simulink model "twa_test"  (R2016a)
settings: Solver=ode8  StartTime=0.0  StopTime=inf  FixedStep=dt  RelTol=1e-3
PreLoadFcn:
  | addpath('d:\Projects\TwistedWireActuator\TWA_parallel_control\init_func')
InitFcn:
  | init_main_twa
  | init_scopes
  | init_twa_homing
  | init_twa_wires
undefined symbols (not defined in the file or in its folder): do_quintic, dt, enc_res_vec, gear_rat_vec, kd_twa, ki_twa, kp_twa, manual_cur, meas_twa_len, N_velocity, pid_mode, pot_volt, q_des, quintic_tf, reset_integ, Signed, vel_filter_coeffs, velmex_pitch, wire_delta, wire_rad
libraries: xpcsensoraylib x4, slrtlib x3, simulink x2, dspswit3 x1
CloseFcn:
  | rtwprivate ssgencode ModelCloseRequest acrochordidae_v1
settings Model: Creator=Roger  LastModifiedBy=ahronoez
settings SolverCC: EnableConcurrentExecution=on
settings DataIOCC: SaveFormat=StructureWithTime  SignalLoggingSaveFormat=ModelDataLogs
settings OptimizationCC: BlockReduction=off  OptimizeBlockIOStorage=off  BufferReuse=off  GlobalBufferReuse=off  ExpressionFolding=off  ExpressionDepthLimit=2147483647  LocalBlockOutputs=off  InitFltsAndDblsToZero=on
settings DebuggingCC: UnderspecifiedInitializationDetection=Classic  MergeDetectMultiDrivingBlocksExec=none  SolverPrmCheckMsg=warning  FcnCallInpInsideContextMsg=UseLocalSettings  StateNameClashWarn=warning
settings HardwareCC: ProdBitPerPointer=32  ProdLargestAtomicFloat=None  ProdWordSize=32  ProdLongLongMode=on  ProdHWDeviceType=Generic->32-bit x86 compatible
settings ModelReferenceCC: PropagateSignalLabelsOutOfModel=off
settings SFSimCC: SimParseCustomCode=off
settings RTWCC: SystemTargetFile=slrt.tlc  TLCOptions=-aSLRTFTZOFF=1  TemplateMakefile=slrt_default_tmf  Description=Simulink Real-Time  GenerateReport=on  RTWCompilerOptimization=Custom  RTWCustomCompilerOptimizations=/arch-IA32
settings SimulinkRealTimeCC: xPCisDownloadable=off
settings ConfigComp: CovModelRefEnable=Off

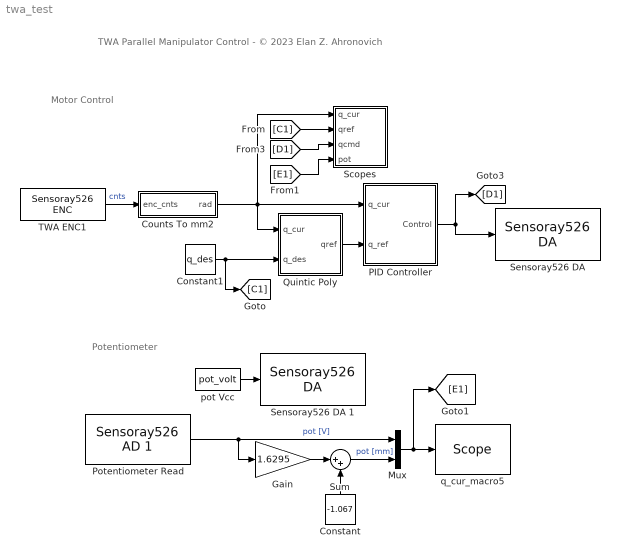
== system twa_test ==
  note: Motor Control
  note: Potentiometer
  note: TWA Parallel Manipulator Control - © 2023 Elan Z. Ahronovich
  Constant : Constant  Value=-1.067
  Constant1 : Constant  Value=q_des
  Counts To mm2 : Subsystem
  Gain : Gain  Gain=1.6295
  Mux : Mux  Inputs=2
  PID Controller : Subsystem
  Potentiometer Read : xpcsensoraylib/A//D/Sensoray526 AD 1  channel=[1]  sampletime=0.001  baseaddress1=0x340  baseaddress2=0
  Quintic Poly : Subsystem
  Scopes : Subsystem
  "Sensoray526 DA " : xpcsensoraylib/D//A/Sensoray526 DA   channel=[4]  reset=[0]  initial=[0]  sampletime=0.001  baseaddress1=0x2c0  baseaddress2=0
  Sensoray526 DA 1 : xpcsensoraylib/D//A/Sensoray526 DA   channel=[2]  reset=[0]  initial=[0]  sampletime=0.001  baseaddress1=0x340  baseaddress2=0
  Sum : Sum  Inputs=|++
  TWA ENC1 : xpcsensoraylib/Encoder/Sensoray526 ENC   channel=4  index=None  resetval=0  initval=0  range=Signed +-2^23  speed=4x  sampletime=dt  baseaddress=0x2c0
  pot Vcc : Constant  Value=pot_volt  SampleTime=-1
  q_cur_macro5 : slrtlib/Displays and Logging/Scope   scopeno=2  scopetype=Target  autostart=on  viewmode=Numerical  formatstr='%0.6f,%0.6f'  grid=on  ylimits=[0,0]  nosamples=125  noprepostsamples=0  interleave=1  triggermode=FreeRun  triggersignal=1  trigsignalfromport=off  triggerlevel=0.0  triggerslope=Either  triggerscope=1  triggersample=0  filename=data.dat  mode=Lazy  writesize=512  autorestart=off  dynamicfilemode=off  maxwritefilesize=512*1024^2
  wires:
  PID Controller/1(Control) -> "Sensoray526 DA "/1, [D1]
  Quintic Poly/1(qref) -> PID Controller/2(q_ref)
  [D1] -> Scopes/3(qcmd)
  TWA ENC1/1 -> Counts To mm2/1(enc_cnts)  "cnts"
  Counts To mm2/1(rad) -> Scopes/1(q_cur), PID Controller/1(q_cur), Quintic Poly/1(q_cur)
  pot Vcc/1 -> Sensoray526 DA 1/1
  Potentiometer Read/1 -> Gain/1, Mux/1  "pot [V]"
  Gain/1 -> Sum/1
  Constant/1 -> Sum/2
  Mux/1 -> [E1], q_cur_macro5/1
  Sum/1 -> Mux/2  "pot [mm]"
  Constant1/1 -> [C1], Quintic Poly/2(q_des)
  [C1] -> Scopes/2(qref)
  [E1] -> Scopes/4(pot)

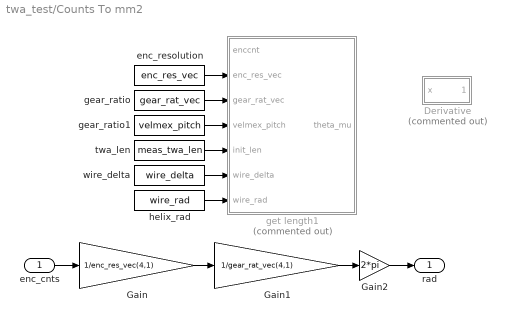
== system twa_test/Counts To mm2 ==
  enc_cnts : Inport
  Derivative : Subsystem  Commented=on
  Gain : Gain  Gain=1/enc_res_vec(4,1)
  Gain1 : Gain  Gain=1/gear_rat_vec(4,1)
  Gain2 : Gain  Gain=2*pi
  enc_resolution : Constant  Value=enc_res_vec  SampleTime=-1
  gear_ratio : Constant  Value=gear_rat_vec  SampleTime=-1
  gear_ratio1 : Constant  Value=velmex_pitch  SampleTime=-1
  get length1 : MATLAB Function  Commented=on  TreatAsAtomicUnit=on
  helix_rad : Constant  Value=wire_rad  SampleTime=-1
  twa_len : Constant  Value=meas_twa_len  SampleTime=-1
  wire_delta : Constant  Value=wire_delta  SampleTime=-1
  rad : Outport
  wires:
  helix_rad/1 -> get length1/7(wire_rad)
  wire_delta/1 -> get length1/6(wire_delta)
  twa_len/1 -> get length1/5(init_len)
  enc_resolution/1 -> get length1/2(enc_res_vec)
  gear_ratio/1 -> get length1/3(gear_rat_vec)
  gear_ratio1/1 -> get length1/4(velmex_pitch)
  Gain/1 -> Gain1/1
  Gain1/1 -> Gain2/1
  enc_cnts/1 -> Gain/1
  Gain2/1 -> rad/1

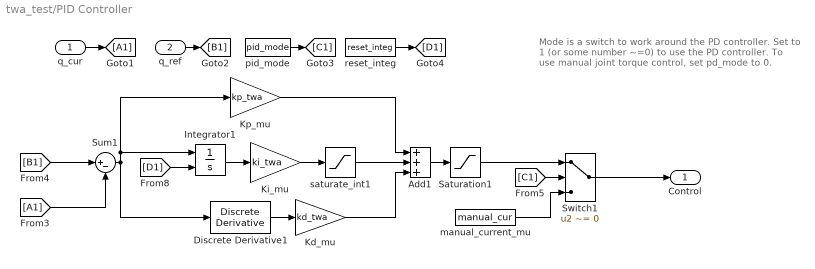
== system twa_test/PID Controller ==
  note: Mode is a switch to work around the PD controller.
      | Set to 1 (or some number ~=0) to use the PD
      | controller. To use manual joint torque control, set
      | pd_mode to 0.
  q_cur : Inport
  q_ref : Inport  Port=2
  Add1 : Sum  Inputs=+++
  Discrete Derivative1 : simulink/Discrete/Discrete Derivative  gainval=1.0  ICPrevScaledInput=0.0  InputProcessing=Inherited  OutMin=[]  OutMax=[]  OutDataType=fixdt(1, 16)  OutScaling=2^-10  DoSatur=off
  Integrator1 : Integrator  ExternalReset=rising
  Kd_mu : Gain  Gain=kd_twa
  Ki_mu : Gain  Gain=ki_twa
  Kp_mu : Gain  Gain=kp_twa
  Saturation1 : Saturate  UpperLimit=5  LowerLimit=-5  LinearizeAsGain=off
  Sum1 : Sum  Inputs=|+-
  Switch1 : Switch  Criteria=u2 ~= 0
  manual_current_mu : Constant  Value=manual_cur  SampleTime=-1
  pid_mode : Constant  Value=pid_mode  SampleTime=-1
  reset_integ : Constant  Value=reset_integ  SampleTime=-1
  saturate_int1 : Saturate  UpperLimit=2.5  LowerLimit=-2.5  LinearizeAsGain=off  SampleTime=dt
  Control : Outport
  wires:
  Kp_mu/1 -> Add1/1
  Kd_mu/1 -> Add1/3
  Add1/1 -> Saturation1/1
  Saturation1/1 -> Switch1/1
  manual_current_mu/1 -> Switch1/3
  Ki_mu/1 -> saturate_int1/1
  saturate_int1/1 -> Add1/2
  Discrete Derivative1/1 -> Kd_mu/1
  Integrator1/1 -> Ki_mu/1
  Sum1/1 -> Kp_mu/1, Integrator1/1, Discrete Derivative1/1
  q_cur/1 -> [A1]
  q_ref/1 -> [B1]
  pid_mode/1 -> [C1]
  [C1] -> Switch1/2
  Switch1/1 -> Control/1
  [B1] -> Sum1/1
  [A1] -> Sum1/2
  reset_integ/1 -> [D1]
  [D1] -> Integrator1/2

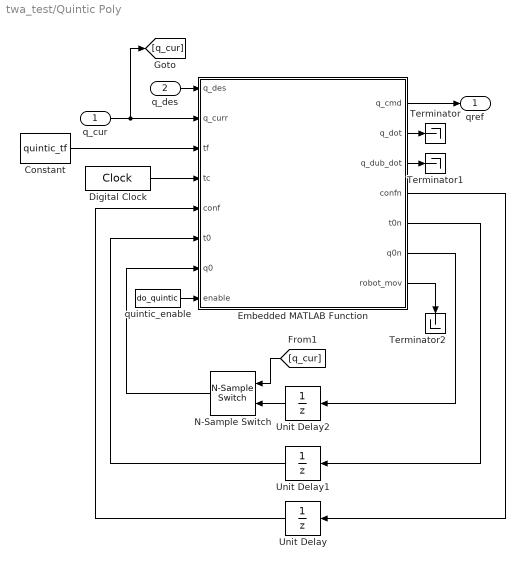
== system twa_test/Quintic Poly ==
  q_cur : Inport
  q_des : Inport  Port=2
  Constant : Constant  Value=quintic_tf  SampleTime=-1
  Digital Clock : DigitalClock  SampleTime=dt
  Embedded MATLAB Function : MATLAB Function  TreatAsAtomicUnit=on
  N-Sample Switch : dspswit3/N-Sample Switch  N=1  reset=off  TriggerType=Rising edge  Ts=dt
  Terminator : Terminator
  Terminator1 : Terminator
  Terminator2 : Terminator
  Unit Delay : UnitDelay  SampleTime=-1
  Unit Delay1 : UnitDelay  SampleTime=-1
  Unit Delay2 : UnitDelay  SampleTime=-1
  quintic_enable : Constant  Value=do_quintic  SampleTime=-1
  qref : Outport
  wires:
  Embedded MATLAB Function/4(confn) -> Unit Delay/1
  Unit Delay/1 -> Embedded MATLAB Function/5(conf)
  Embedded MATLAB Function/5(t0n) -> Unit Delay1/1
  Embedded MATLAB Function/6(q0n) -> Unit Delay2/1
  Unit Delay1/1 -> Embedded MATLAB Function/6(t0)
  Digital Clock/1 -> Embedded MATLAB Function/4(tc)
  q_des/1 -> Embedded MATLAB Function/1(q_des)
  Constant/1 -> Embedded MATLAB Function/3(tf)
  quintic_enable/1 -> Embedded MATLAB Function/8(enable)
  Embedded MATLAB Function/2(q_dot) -> Terminator/1
  Embedded MATLAB Function/3(q_dub_dot) -> Terminator1/1
  N-Sample Switch/1 -> Embedded MATLAB Function/7(q0)
  Unit Delay2/1 -> N-Sample Switch/2
  [q_cur] -> N-Sample Switch/1
  Embedded MATLAB Function/7(robot_mov) -> Terminator2/1
  Embedded MATLAB Function/1(q_cmd) -> qref/1
  q_cur/1 -> Embedded MATLAB Function/2(q_curr), [q_cur]

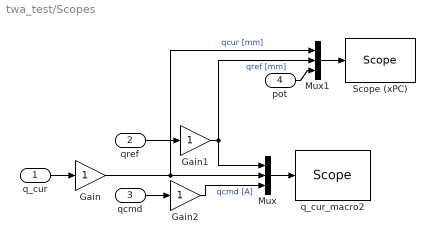
== system twa_test/Scopes ==
  q_cur : Inport
  qref : Inport  Port=2
  qcmd : Inport  Port=3
  pot : Inport  Port=4
  Gain : Gain
  Gain1 : Gain
  Gain2 : Gain
  Mux : Mux  Inputs=3
  Mux1 : Mux  Inputs=3
  "Scope (xPC) " : slrtlib/Displays and Logging/Scope   scopeno=3  scopetype=File  autostart=off  viewmode=Graphical redraw  formatstr='%15.6f'  grid=on  ylimits=[0,0]  nosamples=3  noprepostsamples=0  interleave=1  triggermode=FreeRun  triggersignal=1  trigsignalfromport=off  triggerlevel=0.0  triggerslope=Either  triggerscope=1  triggersample=0  filename=potcal.dat  mode=Lazy  writesize=512  autorestart=on  dynamicfilemode=off  maxwritefilesize=512*1024^2
  q_cur_macro2 : slrtlib/Displays and Logging/Scope   scopeno=1  scopetype=Target  autostart=on  viewmode=Numerical  formatstr='%0.6f, %0.6f, %0.6f'  grid=on  ylimits=[0,0]  nosamples=3  noprepostsamples=0  interleave=1  triggermode=FreeRun  triggersignal=1  trigsignalfromport=off  triggerlevel=0.0  triggerslope=Either  triggerscope=1  triggersample=0  filename=data.dat  mode=Lazy  writesize=512  autorestart=off  dynamicfilemode=off  maxwritefilesize=512*1024^2
  wires:
  q_cur/1 -> Gain/1
  Gain/1 -> Mux1/1, Mux/2  "qcur [mm]"
  qref/1 -> Gain1/1
  Mux/1 -> q_cur_macro2/1
  Gain1/1 -> Mux/1, Mux1/2  "qref [mm]"
  qcmd/1 -> Gain2/1
  Gain2/1 -> Mux/3  "qcmd [A]"
  Mux1/1 -> "Scope (xPC) "/1
  pot/1 -> Mux1/3

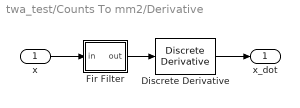
== system twa_test/Counts To mm2/Derivative ==
  x : Inport
  Discrete Derivative : simulink/Discrete/Discrete Derivative  gainval=1.0  ICPrevScaledInput=0.0  InputProcessing=Inherited  OutMin=[]  OutMax=[]  OutDataType=fixdt(1, 16)  OutScaling=2^-10  DoSatur=off
  Fir Filter : Subsystem
  x_dot : Outport
  wires:
  Discrete Derivative/1 -> x_dot/1
  x/1 -> Fir Filter/1(in)
  Fir Filter/1(out) -> Discrete Derivative/1

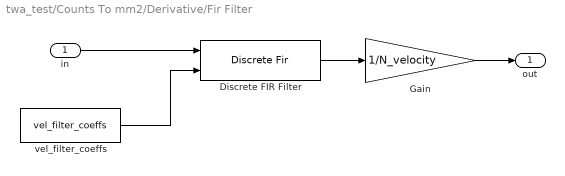
== system twa_test/Counts To mm2/Derivative/Fir Filter ==
  in : Inport
  Discrete FIR Filter : DiscreteFir  CoefSource=Input port  AccumDataTypeStr=Inherit: Same as product output
      settings: InputPortMap=u0,u1
  Gain : Gain  Gain=1/N_velocity
  vel_filter_coeffs : Constant  Value=vel_filter_coeffs  SampleTime=-1
  out : Outport
  wires:
  Discrete FIR Filter/1 -> Gain/1
  vel_filter_coeffs/1 -> Discrete FIR Filter/2
  Gain/1 -> out/1
  in/1 -> Discrete FIR Filter/1

== matlab function twa_test/Counts To mm2/get length1 ==
  data: enccnt input; enc_res_vec input; gear_rat_vec input; velmex_pitch input; init_len input; wire_delta input; wire_rad input; theta_mu output
% this function converts encoder counts to mm
% elan ahronovich 09/2024

function theta_mu = fcn(enccnt,enc_res_vec,gear_rat_vec,velmex_pitch,init_len,wire_delta,wire_rad)

pos_mm = enccnt * (1/enc_res_vec(3,1)) * (1/gear_rat_vec(3,1)) * velmex_pitch;

theta_mu = enccnt * (1/enc_res_vec(4,1)) * (1/gear_rat_vec(4,1)) * 2 * pi;
% 
% if theta_mu <= eps
%     pos_mm = 0;
% else
%     pos_mm = init_len(1,1) - sqrt(init_len(1,1)^2 - (theta_mu*wire_rad)^2);
% end

end

== matlab function twa_test/Quintic Poly/Embedded MATLAB Function ==
  data: q_cmd output; q_des input; q_curr input; tf input; tc input; q_dot output; q_dub_dot output; conf input; confn output; t0 input; t0n output; q0n output; q0 input; enable input; robot_mov output
function [q_cmd,q_dot,q_dub_dot,confn,t0n,q0n,robot_mov] = fifth_order_p(q_des,q_curr,tf,tc,conf,t0,q0,enable)
% number of actuators
n = size(q_des,1);

robot_mov = 0;
eta = q_des - q0;

if enable
    if (eta)'*(eta) > 0
        % conf = 0 means that the 5th order poly
        % is not configured for the desired trajectory.
        % Therefore, the block is initialized.
        if conf == 0               
            q0n = q0;               
            t0n = tc;               
            confn = 1;
            q_cmd = q0;
            q_dot = zeros(n,1);
            q_dub_dot = zeros(n,1);
        else
            q0n = q0;
            t0n = t0;
            confn = conf;
            
            % 5th order polynomial
            a0 = q0;
            a4 = -15*(eta);
            a3 = -2/3 * a4;
            a5 = -2/5 * a4;
            t = tc-t0;
            tau = t/tf;
            
            if t < tf
                robot_mov = 1;
                q_cmd = a0 + a3 * tau^3 + a4 * tau^4 + a5 * tau^5;
                q_dot = 3*a3*t^2/tf^3 + 4*a4*t^3/tf^4 + 5*a5*t^4/tf^5;
                q_dub_dot = 6*a3*t/tf^3 + 12*a4*t^2/tf^4 + 20*a5*t^3/tf^5;
            else
                q_cmd = q_des;
                q_dot = zeros(n,1);
                q_dub_dot = zeros(n,1);
                q0n = q_des;
            end
        end
    else
        q_cmd = q_des;
        q_dot = zeros(n,1);
        q_dub_dot = zeros(n,1);
        confn = 0;
        q0n = q0;
        t0n = t0;
    end
else
    % Configuration space is not used (pdot = 0).
    q_cmd = q_des;
    q_dot = zeros(n,1);
    q_dub_dot = zeros(n,1);       % However we do want to record the current
    confn = 0;                  % position in order to be ready as soon
    t0n = tc;                   % as the enable becomes 1.
    q0n = q_curr;
end
%------------------------------------------------------------------------
